simulink model "Control"  (R2021b)
settings: Solver=VariableStepAuto  StartTime=0.0  StopTime=5  RelTol=1e-3
values from neighbouring files (symbols this model uses):
  kd = 2    [matlab_control.m]
  ki = 0.01    [matlab_control.m]
  kp = 5    [matlab_control.m]
  phiL0 = 0    [matlab_control.m]
  phiR0 = 0    [matlab_control.m]
  theta0 = 0    [Differential_Drive_Demo.m]    (also in matlab_control.m)
  Vd = 1    [matlab_control.m]
  x0 = 0    [Differential_Drive_Demo.m]    (also in matlab_control.m)
  y0 = 0    [Differential_Drive_Demo.m]    (also in matlab_control.m = 0.1)
settings Model: Creator=ANDALIBM  LastModifiedBy=ANDALIBM
settings DataIOCC: ReturnWorkspaceOutputs=off

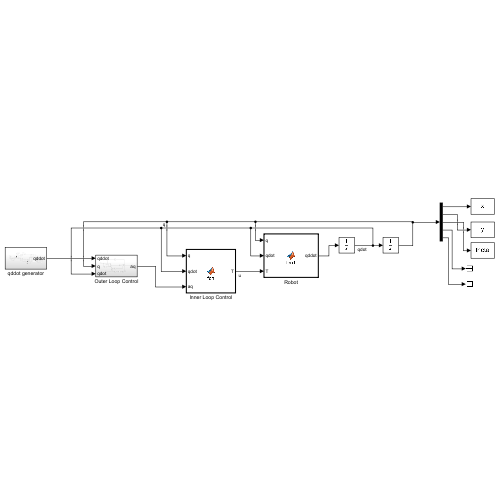
[thumbnail: Simulink's stored preview of the top-level diagram]
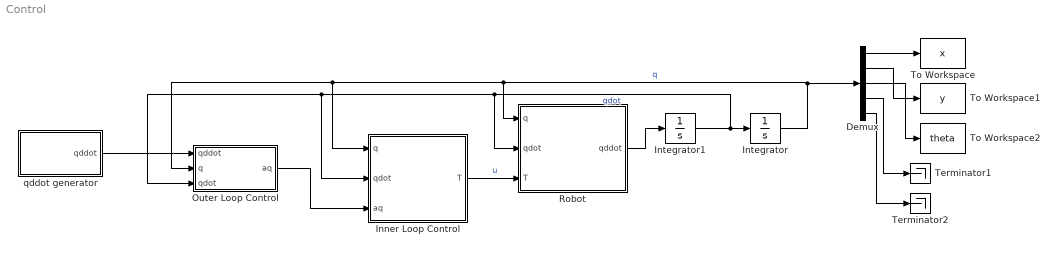
== system Control ==
  Demux : Demux  Outputs=5
  Inner Loop Control : MATLAB Function  TreatAsAtomicUnit=on
  Integrator : Integrator  InitialCondition=[x0;y0;theta0;phiR0;phiL0]
  Integrator1 : Integrator  InitialCondition=[0;0;0;0;0]
  Outer Loop Control : Subsystem
  Robot : MATLAB Function  TreatAsAtomicUnit=on
  Terminator1 : Terminator
  Terminator2 : Terminator
  To Workspace : ToWorkspace  VariableName=x  SampleTime=0.1
  To Workspace1 : ToWorkspace  VariableName=y  SampleTime=0.1
  To Workspace2 : ToWorkspace  VariableName=theta  SampleTime=0.1
  qddot generator : Subsystem
  wires:
  Integrator/1 -> Demux/1, Inner Loop Control/1(q), Outer Loop Control/2(q), Robot/1(q)  "q"
  Robot/1(qddot) -> Integrator1/1
  Integrator1/1 -> Robot/2(qdot), Inner Loop Control/2(qdot), Outer Loop Control/3(qdot), Integrator/1  "qdot"
  Inner Loop Control/1(T) -> Robot/3(T)  "u"
  qddot generator/1(qddot) -> Outer Loop Control/1(qddot)
  Outer Loop Control/1(aq) -> Inner Loop Control/3(aq)
  Demux/1 -> To Workspace/1
  Demux/2 -> To Workspace1/1
  Demux/3 -> To Workspace2/1
  Demux/4 -> Terminator1/1
  Demux/5 -> Terminator2/1

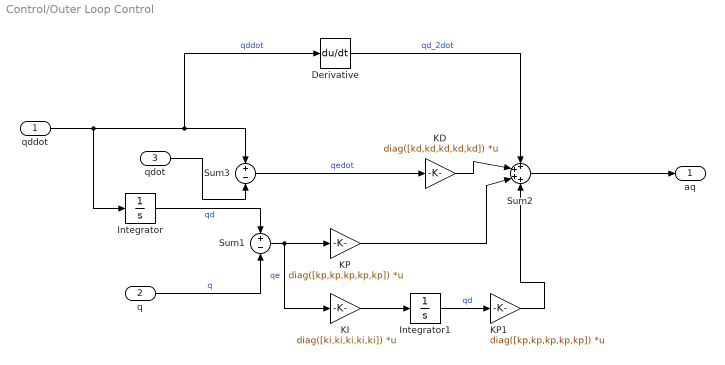
== system Control/Outer Loop Control ==
  qddot : Inport
  q : Inport  Port=2
  qdot : Inport  Port=3
  Derivative : Derivative
  Integrator : Integrator  InitialCondition=[0;0;0;0;0]
  Integrator1 : Integrator  InitialCondition=[0-x0;0-y0;0-theta0;0-phiR0;0-phiL0]
  KD : Gain  Gain=diag([kd,kd,kd,kd,kd])  Multiplication=Matrix(K*u)
  KI : Gain  Gain=diag([ki,ki,ki,ki,ki])  Multiplication=Matrix(K*u)
  KP : Gain  Gain=diag([kp,kp,kp,kp,kp])  Multiplication=Matrix(K*u)
  KP1 : Gain  Gain=diag([kp,kp,kp,kp,kp])  Multiplication=Matrix(K*u)
  Sum1 : Sum  Inputs=+-
  Sum2 : Sum  Inputs=++++
  Sum3 : Sum  Inputs=+-
  aq : Outport
  wires:
  KD/1 -> Sum2/2
  KP/1 -> Sum2/3
  Sum1/1 -> KI/1, KP/1  "qe"
  Sum3/1 -> KD/1  "qedot"
  Sum2/1 -> aq/1
  qddot/1 -> Integrator/1, Derivative/1, Sum3/1  "qddot"
  Integrator/1 -> Sum1/1  "qd"
  q/1 -> Sum1/2  "q"
  qdot/1 -> Sum3/2
  Derivative/1 -> Sum2/1  "qd_2dot"
  Integrator1/1 -> KP1/1  "qd"
  KP1/1 -> Sum2/4
  KI/1 -> Integrator1/1

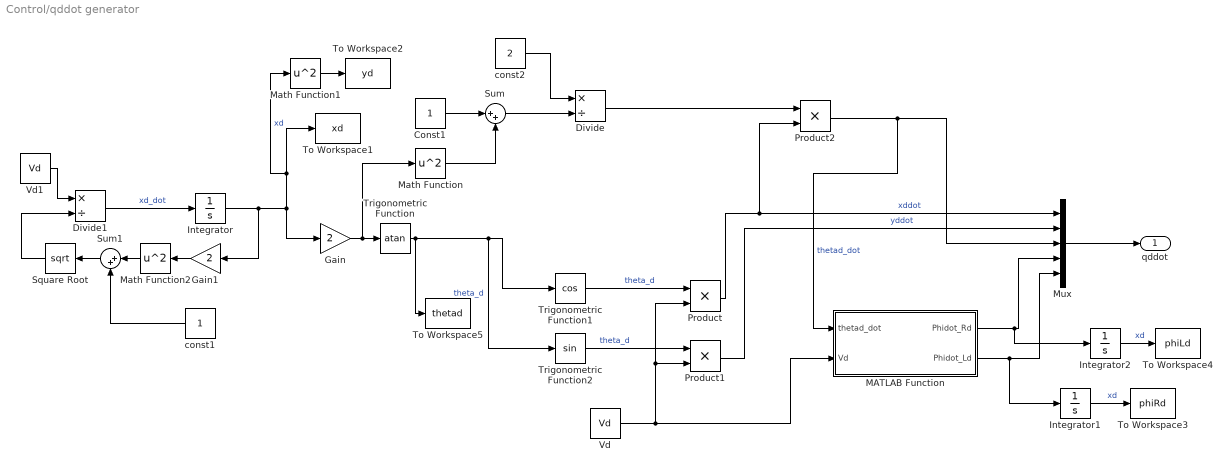
== system Control/qddot generator ==
  Const1 : Constant
  Divide : Product  Inputs=*/
  Divide1 : Product  Inputs=*/
  Gain : Gain  Gain=2
  Gain1 : Gain  Gain=2
  Integrator : Integrator
  Integrator1 : Integrator
  Integrator2 : Integrator
  MATLAB Function : MATLAB Function  TreatAsAtomicUnit=on
  Math Function : Math  Operator=square  SaturateOnIntegerOverflow=on
  Math Function1 : Math  Operator=square  SaturateOnIntegerOverflow=on
  Math Function2 : Math  Operator=square  SaturateOnIntegerOverflow=on
  Mux : Mux  Inputs=5
  Product : Product
  Product1 : Product
  Product2 : Product
  Square Root : Sqrt  SaturateOnIntegerOverflow=on
  Sum : Sum  Inputs=|++
  Sum1 : Sum  Inputs=|++
  To Workspace1 : ToWorkspace  VariableName=xd  SampleTime=0.1
  To Workspace2 : ToWorkspace  VariableName=yd  SampleTime=0.1
  To Workspace3 : ToWorkspace  VariableName=phiRd  SampleTime=0.1
  To Workspace4 : ToWorkspace  VariableName=phiLd  SampleTime=0.1
  To Workspace5 : ToWorkspace  VariableName=thetad  SampleTime=0.1
  Trigonometric Function : Trigonometry  Operator=atan
  Trigonometric Function1 : Trigonometry  Operator=cos
  Trigonometric Function2 : Trigonometry
  Vd : Constant  Value=Vd
  Vd1 : Constant  Value=Vd
  const1 : Constant
  const2 : Constant  Value=2
  qddot : Outport
  wires:
  Gain/1 -> Math Function/1, Trigonometric Function/1
  Trigonometric Function/1 -> To Workspace5/1, Trigonometric Function2/1, Trigonometric Function1/1  "theta_d"
  Trigonometric Function1/1 -> Product/1  "theta_d"
  Trigonometric Function2/1 -> Product1/1  "theta_d"
  Vd/1 -> MATLAB Function/2(Vd), Product1/2, Product/2
  Mux/1 -> qddot/1
  Product/1 -> Product2/2, Mux/1  "xddot"
  Product1/1 -> Mux/2  "yddot"
  Const1/1 -> Sum/1
  Math Function/1 -> Sum/2
  Product2/1 -> MATLAB Function/1(thetad_dot), Mux/3  "thetad_dot"
  Sum/1 -> Divide/2
  const2/1 -> Divide/1
  Divide/1 -> Product2/1
  MATLAB Function/1(Phidot_Rd) -> Integrator2/1, Mux/4
  MATLAB Function/2(Phidot_Ld) -> Integrator1/1, Mux/5
  Math Function1/1 -> To Workspace2/1
  Integrator/1 -> Gain/1, Math Function1/1, To Workspace1/1, Gain1/1  "xd"
  Gain1/1 -> Math Function2/1
  Math Function2/1 -> Sum1/1
  const1/1 -> Sum1/2
  Vd1/1 -> Divide1/1
  Square Root/1 -> Divide1/2
  Sum1/1 -> Square Root/1
  Divide1/1 -> Integrator/1  "xd_dot"
  Integrator1/1 -> To Workspace3/1  "xd"
  Integrator2/1 -> To Workspace4/1  "xd"

== matlab function Control/Robot ==
  data: q input; qddot output; qdot input; T input
function qddot  = fcn1(q,qdot,T)

theta=q(3);
thetadot=qdot(3);

% parameters
mB=2;
mW=0.05;
W=0.15;
R=0.06;
t=0.01;
d=0;

Iyy=mW*R^2/2;
Izz=mW*(3*R^2+t^2)/12;
IB=0.0225;

mT=mB+2*mW;
IT=IB+2*mW*W^2+2*Izz;

C=[1 0 0 R*cos(theta)/2 -R*cos(theta)/2;
   0 1 0 R*sin(theta)/2 -R*sin(theta)/2;
   0 0 1 0.5*R/W         0.5*R/W];

Cdot=[0 0 0 -R*sin(theta)*thetadot/2    R*sin(theta)*thetadot/2;
      0 0 0  R*cos(theta)*thetadot/2   -R*cos(theta)*thetadot/2;
      0 0 0  0                          0];

M=[mT                      0          -mB*d*sin(theta) 0  0;
   0                       mT          mB*d*cos(theta) 0  0;
   -mB*d*sin(theta)  mB*d*cos(theta)         IT        0  0;
   0                       0                 0        Iyy 0;
   0                       0                 0        0 Iyy];

B=-mB*d*(thetadot^2)*[cos(theta);sin(theta);0;0;0];

lambda=-inv(C*inv(M)*C')*(C*inv(M)*(T-B)+Cdot*qdot);

qddot=inv(M)*(T+C'*lambda-B);

== matlab function Control/Inner Loop Control ==
  data: q input; T output; qdot input; aq input
function T = fcn(q, qdot, aq)

theta=q(3);
thetadot=qdot(3);

% parameters
mB=2;
mW=0.05;
W=0.15;
R=0.06;
t=0.01;
d=0;

Iyy=mW*R^2/2;
Izz=mW*(3*R^2+t^2)/12;
IB=0.0225;

mT=mB+2*mW;
IT=IB+2*mW*W^2+2*Izz;

C=[1 0 0 R*cos(theta)/2 -R*cos(theta)/2;
   0 1 0 R*sin(theta)/2 -R*sin(theta)/2;
   0 0 1 0.5*R/W         0.5*R/W];

Cdot=[0 0 0 -R*sin(theta)*thetadot/2    R*sin(theta)*thetadot/2;
      0 0 0  R*cos(theta)*thetadot/2   -R*cos(theta)*thetadot/2;
      0 0 0  0                          0];

M=[mT                      0          -mB*d*sin(theta) 0  0;
   0                       mT          mB*d*cos(theta) 0  0;
   -mB*d*sin(theta)  mB*d*cos(theta)         IT        0  0;
   0                       0                 0        Iyy 0;
   0                       0                 0        0 Iyy];

B=-mB*d*(thetadot^2)*[cos(theta);sin(theta);0;0;0];

Ap=-inv(C*inv(M)*C');
A=-inv(C*inv(M)*C')*C*inv(M);

T=inv(eye(5,5)-C'*A)*(M*aq+B-C'*A*B+C'*Ap*Cdot*qdot);

== matlab function Control/qddot generator/MATLAB Function ==
  data: thetad_dot input; Phidot_Rd output; Phidot_Ld output; Vd input
function [Phidot_Rd,Phidot_Ld] = fcn(thetad_dot,Vd)

R=0.06;
L=0.3;

A=[R/2 +R/2;R/L -R/L];

temp=inv(A)*[Vd;thetad_dot];

Phidot_Rd=-temp(1);
Phidot_Ld=temp(2);
